simulink model "untitled"  (Simulink 6.6)
settings: Solver=ode45  StartTime=0.0  StopTime=10.0  MaxStep=0.001  RelTol=1e-3
libraries: simulink x1
settings Model: Creator=student  LastModifiedBy=student

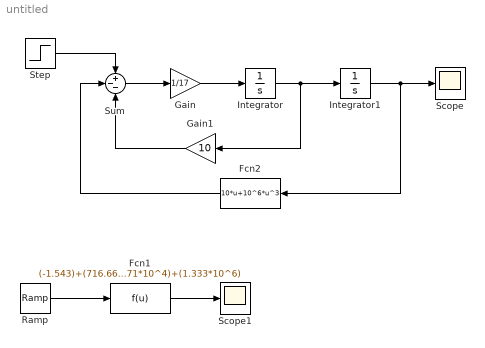
== system untitled ==
  Fcn1 : Fcn  Expr=(-1.543)+(716.667)+(4.071*10^4)+(1.333*10^6)
  Fcn2 : Fcn  Orientation=left  Expr=10*u+10^6*u^3
  Gain : Gain  Gain=1/17
  Gain1 : Gain  Orientation=left  Gain=10
  Integrator : Integrator
  Integrator1 : Integrator
  Ramp : simulink/Sources/Ramp  SystemSampleTime=-1  slope=0.004  start=0  X0=-0.02
  Scope : Scope
      settings: TimeRange=0.006144393241168444  YMin=-1.09878e+006  YMax=-1.0982e+006
  Scope1 : Scope
      settings: TimeRange=0.006144393241168444  YMin=0.00387701298701299  YMax=0.00579701298701299
  Step : Step  Time=0  Before=1  After=100  SampleTime=0
  Sum : Sum  Inputs=+--
  wires:
  Step/1 -> Sum/1
  Sum/1 -> Gain/1
  Gain/1 -> Integrator/1
  Integrator/1 -> Integrator1/1, Gain1/1
  Integrator1/1 -> Scope/1, Fcn2/1
  Gain1/1 -> Sum/3
  Fcn2/1 -> Sum/2
  Ramp/1 -> Fcn1/1
  Fcn1/1 -> Scope1/1
